simulink model "F"  (R2016b)
settings: Solver=VariableStepAuto  StartTime=0.0  StopTime=10  RelTol=1e-3
libraries: fuzblock x3, simulink x2
settings Model: Creator=Mohammad  LastModifiedBy=Mohammad
settings SolverCC: ZeroCrossControl=DisableAll

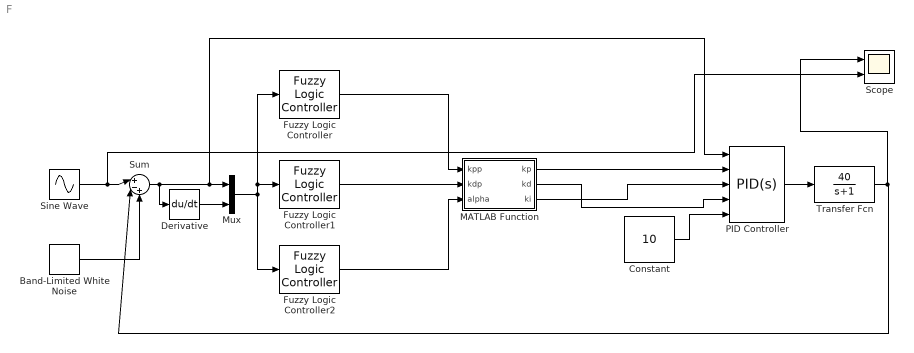
== system F ==
  Band-Limited White Noise : simulink/Sources/Band-Limited White Noise  Cov=[0.1]  Ts=0.1  seed=[23341]
  Constant : Constant  Value=10
  Derivative : Derivative
  Fuzzy Logic Controller : fuzblock/Fuzzy Logic  Controller  fis='FKP.fis'
  Fuzzy Logic Controller1 : fuzblock/Fuzzy Logic  Controller  fis='FKD.fis'
  Fuzzy Logic Controller2 : fuzblock/Fuzzy Logic  Controller  fis='fu.fis'
  MATLAB Function : MATLAB Function  TreatAsAtomicUnit=on
  Mux : Mux  Inputs=2
  PID Controller : simulink/Continuous/PID Controller  Controller=PID  TimeDomain=Continuous-time  SampleTime=-1  IntegratorMethod=Forward Euler  FilterMethod=Forward Euler  Form=Parallel  UseFilter=on  ControllerParametersSource=external  P=1  I=1  D=0  N=100  InitialConditionSource=internal  InitialConditionForIntegrator=0  InitialConditionForFilter=0  ExternalReset=none  ZeroCross=off  LimitOutput=off  UpperSaturationLimit=inf  LowerSaturationLimit=-inf  LinearizeAsGain=on  AntiWindupMode=none  Kb=1  TrackingMode=off  Kt=1  PParamMin=[]  PParamMax=[]  IParamMin=[]  IParamMax=[]  DParamMin=[]  DParamMax=[]  NParamMin=[]  NParamMax=[]  KbParamMin=[]  KbParamMax=[]  KtParamMin=[]  KtParamMax=[]  POutMin=[]  POutMax=[]  IOutMin=[]  IOutMax=[]  DOutMin=[]  DOutMax=[]  NOutMin=[]  NOutMax=[]  KbOutMin=[]  KbOutMax=[]  KtOutMin=[]  KtOutMax=[]  IntegratorOutMin=[]  IntegratorOutMax=[]  FilterOutMin=[]  FilterOutMax=[]  SumOutMin=[]  SumOutMax=[]  SumI1OutMin=[]  SumI1OutMax=[]  SumI2OutMin=[]  SumI2OutMax=[]  SumI3OutMin=[]  SumI3OutMax=[]  SumDOutMin=[]  SumDOutMax=[]  SaturationOutMin=[]  SaturationOutMax=[]  IntegratorContinuousStateAttributes=''  IntegratorStateMustResolveToSignalObject=off  IntegratorRTWStateStorageClass=Auto  FilterContinuousStateAttributes=''  FilterStateMustResolveToSignalObject=off  FilterRTWStateStorageClass=Auto  DifferentiatorICPrevScaledInput=0  DifferentiatorOutMin=[]  DifferentiatorOutMax=[]
  Scope : Scope  NumInputPorts=2
  Sine Wave : Sin  SampleTime=0
  Sum : Sum  Inputs=|+-+
  Transfer Fcn : TransferFcn  Numerator=[40]  Denominator=[1 1]
  wires:
  Fuzzy Logic Controller/1 -> MATLAB Function/1(kpp)
  Fuzzy Logic Controller1/1 -> MATLAB Function/2(kdp)
  Fuzzy Logic Controller2/1 -> MATLAB Function/3(alpha)
  MATLAB Function/1(kp) -> PID Controller/2
  PID Controller/1 -> Transfer Fcn/1
  Transfer Fcn/1 -> Scope/1, Sum/2
  Sine Wave/1 -> Scope/2, Sum/1
  Sum/1 -> Derivative/1, PID Controller/1, Mux/1
  Derivative/1 -> Mux/2
  Mux/1 -> Fuzzy Logic Controller2/1, Fuzzy Logic Controller/1, Fuzzy Logic Controller1/1
  Constant/1 -> PID Controller/5
  MATLAB Function/3(ki) -> PID Controller/3
  MATLAB Function/2(kd) -> PID Controller/4
  Band-Limited White Noise/1 -> Sum/3

== matlab function F/MATLAB Function ==
  data: kpp input; kp output; kdp input; alpha input; kd output; ki output
function [kp,kd,ki] = G(kpp,kdp,alpha)
kp=5*(kpp)
kd=5*(kdp)
ki=kp*kp/(alpha*kd)
ti=alpha*kp/ki;
